simulink subsystem "Subsystem_3S"  (R2025b)
settings: Solver=VariableStepAuto  StartTime=0.0  StopTime=10.0  RelTol=1e-3
model mask{Waterlevel_1=275, Height=1, Max_cap_1=300, Diameter=24.5, K=7.77*1e-5, A=0.0117, B=0.1252, Duration_S1=10, Flowrate_S1=1, BurstStart=1, BurstFlow=1, BurstDur=1, RainSwitch_S1=on, Waterlevel_2=150, Height_2=1, Max_cap_2=300, Diameter_2=24.5, K_2=7.77*1e-5, A_2=0.0117, B_2=0.1252, Duration_2=10, Flowrate_2=1, BurstStart_2=1, BurstFlow_2=1, BurstDur_2=1, RainSwitch_S2=on, InitialCondition=275, Height_3=1, Max_cap_3=300, Diameter_3=24.5, K_3=7.77*1e-5, A_3=0.0117, B_3=0.1252, Duration_3=60, Flowrate_3=5, BurstStart_3=60, BurstFlow_3=20, BurstDur_3=60, RainSwitch_S3=on, DelayLength=0, rain_start=0, station_order=0, flip_order=off, EnableBurst=on}
  mask prompts: Waterlevel_1 "Initial water level:"; Max_cap_1 "Max capacity:"; A "Valve coeff A:"; Duration_S1 "Duration (sec):"; Flowrate_S1 "Flowrate (liters/min):"; BurstStart "Burst start:"; BurstFlow "Burst flow:"; BurstDur "Burst duration:"; RainSwitch_S1 "Set rain on/off"; Waterlevel_2 "Initial water level:"; Height_2 "Height:"; Max_cap_2 "Max capacity:"; Diameter_2 "Diameter:"; K_2 "K:"; A_2 "Valve coeff A:"; B_2 "B:"; Duration_2 "Duration (sec):"; Flowrate_2 "Flowrate (liters/min):"; BurstStart_2 "Burst start:"; BurstFlow_2 "Burst flow:"; BurstDur_2 "Burst duration:"; RainSwitch_S2 "Set rain on/off"; InitialCondition "Initial level:"; Height_3 "Height:"; Max_cap_3 "Max capacity:"; Diameter_3 "Diameter:"; K_3 "K:"; A_3 "Valve coeff A:"; B_3 "B:"; Duration_3 "Duration"; Flowrate_3 "Flowrate (liters/min)"; BurstStart_3 "Burst start:"; BurstFlow_3 "Burst flow:"; BurstDur_3 "Burst duration:"; RainSwitch_S3 "Set rain on/off"; DelayLength "Transport delay(sec):"; rain_start "Rain start (sec):"; station_order "Station order:"; flip_order "Flip order"; EnableBurst "Enable cloud burst"
settings Model: Creator=klump  LastModifiedBy=klump

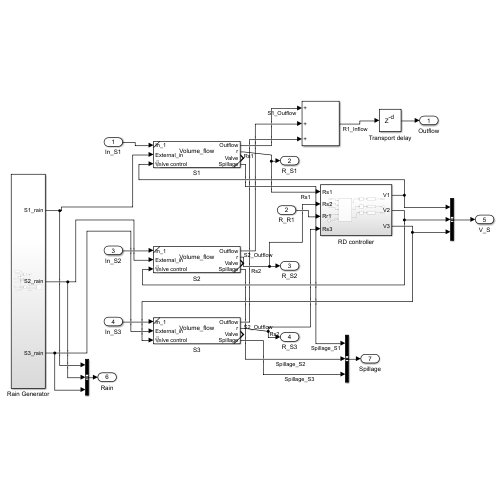
[thumbnail: Simulink's stored preview of the top-level diagram]
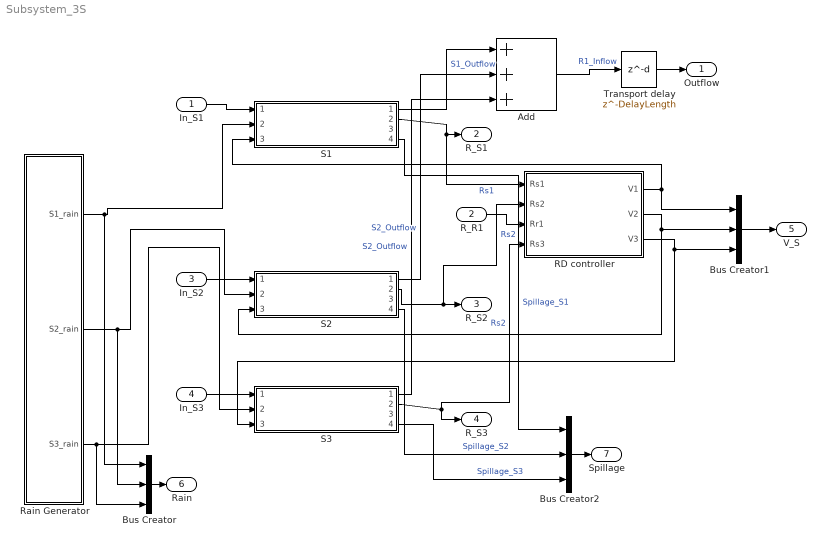
== system Subsystem_3S ==
  In_S1 : Inport
  R_R1 : Inport  Port=2
  In_S2 : Inport  Port=3
  In_S3 : Inport  Port=4
  Add : Sum  Inputs=+++
  Bus Creator : BusCreator  Inputs=3
  Bus Creator1 : BusCreator  Inputs=3
  Bus Creator2 : BusCreator  Inputs=3
  RD controller : Subsystem
  Rain Generator : Subsystem
  S1 : Subsystem  ReferencedSubsystem=Volume_flow  InitialCondition=Waterlevel_1  Max_cap=Max_cap_1  Diameter=Diameter  K=K  Height=Height  A=A  B=B
  S2 : Subsystem  ReferencedSubsystem=Volume_flow  InitialCondition=Waterlevel_2  Max_cap=Max_cap_2  Diameter=Diameter_2  K=K_2  Height=Height_2  A=A_2  B=B_2
  S3 : Subsystem  ReferencedSubsystem=Volume_flow  InitialCondition=InitialCondition  Max_cap=Max_cap_3  Diameter=Diameter_3  K=K_3  Height=Height_3  A=A_3  B=B_3
  Transport delay : Delay  DelayLength=DelayLength  InputProcessing=Columns as channels (frame based)
  Outflow : Outport
  R_S1 : Outport  Port=2
  R_S2 : Outport  Port=3
  R_S3 : Outport  Port=4
  V_S : Outport  Port=5
  Rain : Outport  Port=6
  Spillage : Outport  Port=7
  wires:
  In_S2/1 -> S2/1
  R_R1/1 -> RD controller/3(Rr1)
  S2/2 -> R_S2/1, RD controller/2(Rs2)  "Rs2"
  RD controller/2(V2) -> S2/3, Bus Creator1/2
  Bus Creator1/1 -> V_S/1
  Add/1 -> Transport delay/1  "R1_Inflow"
  Transport delay/1 -> Outflow/1
  S2/1 -> Add/2  "S2_Outflow"
  S1/2 -> R_S1/1, RD controller/1(Rs1)  "Rs1"
  S1/1 -> Add/1  "S1_Outflow"
  RD controller/1(V1) -> S1/3, Bus Creator1/1
  Rain Generator/1(S1_rain) -> S1/2, Bus Creator/1
  In_S1/1 -> S1/1
  Rain Generator/2(S2_rain) -> S2/2, Bus Creator/2
  S3/1 -> Add/3  "S2_Outflow"
  In_S3/1 -> S3/1
  Rain Generator/3(S3_rain) -> S3/2, Bus Creator/3
  RD controller/3(V3) -> Bus Creator1/3, S3/3
  S3/2 -> R_S3/1, RD controller/4(Rs3)  "Rs2"
  Bus Creator/1 -> Rain/1
  Bus Creator2/1 -> Spillage/1
  S1/4 -> Bus Creator2/1  "Spillage_S1"
  S2/4 -> Bus Creator2/2  "Spillage_S2"
  S3/4 -> Bus Creator2/3  "Spillage_S3"

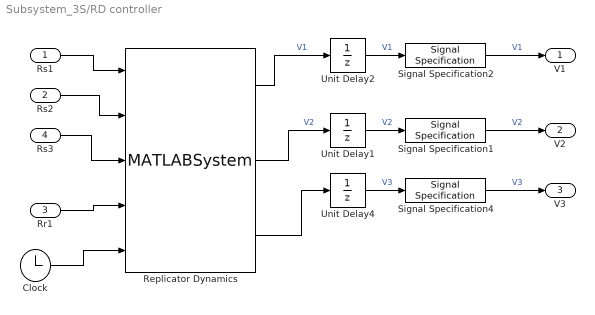
== system Subsystem_3S/RD controller ==
  Rs1 : Inport
  Rs2 : Inport  Port=2
  Rr1 : Inport  Port=3
  Rs3 : Inport  Port=4
  Clock : Clock
  Replicator Dynamics : MATLABSystem  System=RD_controller_3S  SimulateUsing=Code generation
      mask Type: RD_controller_3S
  Signal Specification1 : SignalSpecification  Dimensions=1
  Signal Specification2 : SignalSpecification  Dimensions=1
  Signal Specification4 : SignalSpecification  Dimensions=1
  Unit Delay1 : UnitDelay  SampleTime=-1  HasFrameUpgradeWarning=on
  Unit Delay2 : UnitDelay  SampleTime=-1  HasFrameUpgradeWarning=on
  Unit Delay4 : UnitDelay  SampleTime=-1  HasFrameUpgradeWarning=on
  V1 : Outport
  V2 : Outport  Port=2
  V3 : Outport  Port=3
  wires:
  Rr1/1 -> Replicator Dynamics/4
  Rs2/1 -> Replicator Dynamics/2
  Rs1/1 -> Replicator Dynamics/1
  Clock/1 -> Replicator Dynamics/5
  Unit Delay2/1 -> Signal Specification2/1  "V1"
  Signal Specification2/1 -> V1/1  "V1"
  Unit Delay1/1 -> Signal Specification1/1  "V2"
  Signal Specification1/1 -> V2/1  "V2"
  Replicator Dynamics/2 -> Unit Delay1/1  "V2"
  Replicator Dynamics/1 -> Unit Delay2/1  "V1"
  Signal Specification4/1 -> V3/1  "V3"
  Unit Delay4/1 -> Signal Specification4/1  "V3"
  Rs3/1 -> Replicator Dynamics/3
  Replicator Dynamics/3 -> Unit Delay4/1

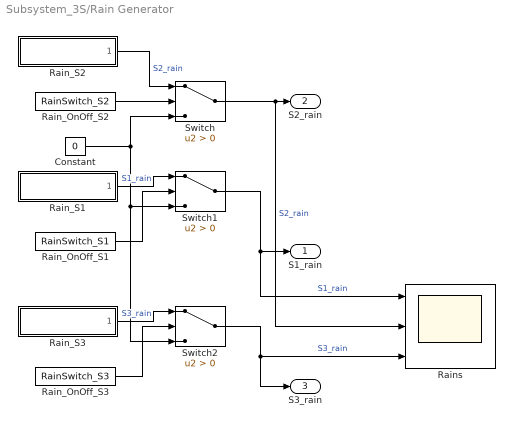
== system Subsystem_3S/Rain Generator ==
  Constant : Constant  Value=0
  Rain_OnOff_S1 : Constant  Value=RainSwitch_S1
  Rain_OnOff_S2 : Constant  Value=RainSwitch_S2
  Rain_OnOff_S3 : Constant  Value=RainSwitch_S3
  Rain_S1 : Subsystem  ReferencedSubsystem=Rain  Duration=Duration_S1  Flowrate=Flowrate_S1  BurstStart=BurstStart  BurstFlow=BurstFlow  BurstDur=BurstDur  flip_order=off  rain_start=rain_start  station_order=station_order  EnableBurst=on
  Rain_S2 : Subsystem  ReferencedSubsystem=Rain  Duration=Duration_2  Flowrate=Flowrate_2  BurstStart=BurstStart_2  BurstFlow=BurstFlow_2  BurstDur=BurstDur_2  flip_order=off  rain_start=rain_start  station_order=station_order  EnableBurst=on
  Rain_S3 : Subsystem  ReferencedSubsystem=Rain  Duration=Duration_3  Flowrate=Flowrate_3  BurstStart=BurstStart_3  BurstFlow=BurstFlow_3  BurstDur=BurstDur_3  flip_order=off  rain_start=rain_start  station_order=station_order  EnableBurst=on
  Rains : Scope  NumInputPorts=3
      settings: ActiveDisplayYMinimum=-1  ActiveDisplayYMaximum=1  DataLoggingVariableName=ScopeData2
  Switch : Switch  Criteria=u2 > Threshold  SaturateOnIntegerOverflow=off  InputSameDT=off
  Switch1 : Switch  Criteria=u2 > Threshold  SaturateOnIntegerOverflow=off  InputSameDT=off
  Switch2 : Switch  Criteria=u2 > Threshold  SaturateOnIntegerOverflow=off  InputSameDT=off
  S1_rain : Outport
  S2_rain : Outport  Port=2
  S3_rain : Outport  Port=3
  wires:
  Rain_OnOff_S1/1 -> Switch1/2
  Rain_S2/1 -> Switch/1  "S2_rain"
  Rain_S1/1 -> Switch1/1  "S1_rain"
  Switch1/1 -> S1_rain/1, Rains/1  "S1_rain"
  Rain_OnOff_S2/1 -> Switch/2
  Switch/1 -> S2_rain/1, Rains/2  "S2_rain"
  Rain_OnOff_S3/1 -> Switch2/2
  Rain_S3/1 -> Switch2/1  "S3_rain"
  Switch2/1 -> Rains/3, S3_rain/1  "S3_rain"
  Constant/1 -> Switch2/3, Switch1/3, Switch/3
